simulink model "all_together_simu_v2"  (R2020b)
settings: Solver=FixedStepDiscrete  StartTime=0.0  StopTime=simTime  RelTol=1e-3
InitFcn:
  | setup
values from neighbouring files (symbols this model uses):
  COLS = 752    [setup.m]    (also in setup_old.m = 640)
  Hh = abs(V(:,1)'*sqrt(S(1,1)))    [setup_old.m]
  Hv = abs(U(:,1)*sqrt(S(1,1)))    [setup_old.m]
undefined symbols (not defined in the file or in its folder): gray, Rec, SDTV
libraries: hdlsllib x52, visionhdlio x7, visionsinks x3, simulink x2, visionconversions x1, visionsources x1
(part 1 of 2)
settings Model: DataTypeOverride=Off  SimulationMode=accelerator  Creator=The MathWorks, Inc.  LastModifiedBy=Ethan
settings SolverCC: AutoInsertRateTranBlk=on
settings DataIOCC: LimitDataPoints=on  SaveOutput=off  SignalLogging=off  SaveTime=off  ReturnWorkspaceOutputs=off
settings OptimizationCC: BlockReduction=off  ConditionallyExecuteInputs=off  DefaultParameterBehavior=Inlined  LifeSpan=inf
settings DebuggingCC: AlgebraicLoopMsg=error  SingleTaskRateTransMsg=error  ParameterPrecisionLossMsg=none  AllowSymbolicDim=off  StrictBusMsg=ErrorOnBusTreatedAsVector  SFUnexpectedBacktrackingDiag=warning  SFNoUnconditionalDefaultTransitionDiag=warning  SFExecutionAtInitializationDiag=none  ArithmeticOperatorsInVariantConditions=warning
settings HardwareCC: ProdBitPerPointer=32  ProdBitPerSizeT=32  ProdBitPerPtrDiffT=32  ProdLargestAtomicFloat=None  ProdIntDivRoundTo=Undefined  ProdEndianess=Unspecified  ProdWordSize=32  ProdHWDeviceType=ASIC/FPGA->ASIC/FPGA  ProdEqTarget=off
settings SFSimCC: SimUseLocalCustomCode=off  CustomCodeUndefinedFunction=UseInterfaceOnly
settings RTWCC: RTWUseLocalCustomCode=off
settings CodeAppCC: StateflowObjectComments=on
settings GRTTargetCC: TargetLangStandard=C89/C90 (ANSI)
settings ConfigComp: CovMetricSettings=dw  CovSaveCumulativeToWorkspaceVar=on  CovSaveSingleToWorkspaceVar=on  CovExternalEMLEnable=off  CovSFcnEnable=off

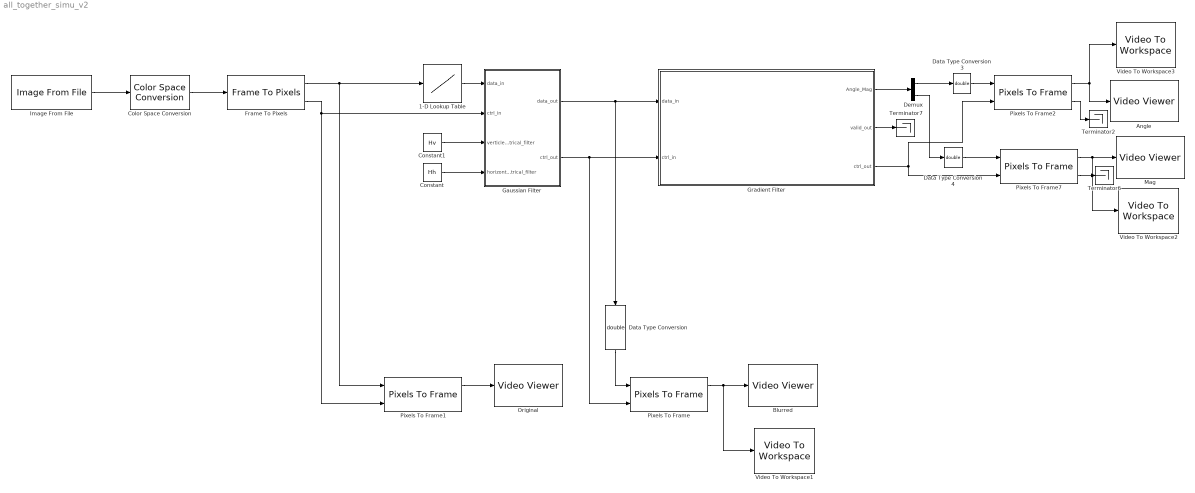
== system all_together_simu_v2 ==
  1-D Lookup Table : Lookup_n-D  NumberOfTableDimensions=1  BreakpointsForDimension1=[0:255]  Table=[0:1/255:1]  ExtrapMethod=Clip  InternalRulePriority=Speed  OutDataTypeStr=fixdt(0,16,15)  RndMeth=Simplest  InputSameDT=on
  Angle : VideoViewer  colormapValue=gray(256)  FigPos=[1922 517 909 409]
  Blurred : VideoViewer  FigPos=[951 815 859 624]
  Color Space Conversion : visionconversions/Color Space  Conversion  conversion=Obsolete  conversionActive=R'G'B' to intensity  wp_str=D65  rec=Rec. 601 (SDTV)  sys=1125/60/2:1  imagePorts=One multidimensional signal
  Constant : Constant  Value=Hh  OutDataTypeStr=Inherit: Inherit via back propagation  SampleTime=-1
  Constant1 : Constant  Value=Hv  OutDataTypeStr=Inherit: Inherit via back propagation  SampleTime=-1
  Data Type Conversion : DataTypeConversion  OutDataTypeStr=double
  Data Type Conversion3 : DataTypeConversion  OutDataTypeStr=double
  Data Type Conversion4 : DataTypeConversion  OutDataTypeStr=double
  Demux : Demux  Outputs=2
  Frame To Pixels : visionhdlio/Frame To Pixels  NumComponents=1  NumPixels=1  VideoFormat=480p  ActivePixelsPerLine=32  ActiveVideoLines=18  TotalPixelsPerLine=42  TotalVideoLines=28  StartingActiveLine=6  FrontPorch=5  SampleTime=0
      settings: SourceProductName=Vision HDL Toolbox
  Gaussian Filter : Subsystem
  Gradient Filter : Subsystem
  Image From File : visionsources/Image From File  Tag=vipblks_nd  FileName=..\..\visualStudio\images\input\start.png  Ts=1  imagePorts=One multidimensional signal  OutPortLabels=R|G|B  ImageDataType=uint8  sdImageDataType=uint(8)  Signed=on  WordLength=16  FractionLengthMode=User-defined  FractionLength=15
  Mag : VideoViewer  FigPos=[1914 1017 954 411]
  Original : VideoViewer  FigPos=[946 1004 813 538]
  Pixels To Frame{,1..2,7} (4 alike) : visionhdlio/Pixels To Frame  NumComponents=1  NumPixels=1  VideoFormat=480p  ActivePixelsPerLine=32  ActiveVideoLines=18  TotalPixelsPerLine=42  TotalVideoLines=28
      settings: SourceProductBaseCode=VT
  Terminator2 : Terminator
  Terminator6 : Terminator
  Terminator7 : Terminator
  Video To Workspace1 : visionsinks/Video To Workspace  VariableName=gaussian  NumInputs=1  DataLimit=10  DecimationFactor=1  LogFi=off  InPortLabels=R|G|B
      settings: SourceProductBaseCode=VP
  Video To Workspace2 : visionsinks/Video To Workspace  VariableName=mag  NumInputs=1  DataLimit=10  DecimationFactor=1  LogFi=off  InPortLabels=R|G|B
      settings: SourceProductBaseCode=VP
  Video To Workspace3 : visionsinks/Video To Workspace  VariableName=angle  NumInputs=1  DataLimit=10  DecimationFactor=1  LogFi=off  InPortLabels=R|G|B
      settings: SourceProductBaseCode=VP
  wires:
  Frame To Pixels/2 -> Pixels To Frame1/2, Gaussian Filter/2(ctrl_in)
  Image From File/1 -> Color Space Conversion/1
  Constant/1 -> Gaussian Filter/4(horizontal_symmetrical_filter)
  Constant1/1 -> Gaussian Filter/3(verticle_symmetrical_filter)
  1-D Lookup Table/1 -> Gaussian Filter/1(data_in)
  Color Space Conversion/1 -> Frame To Pixels/1
  Frame To Pixels/1 -> 1-D Lookup Table/1, Pixels To Frame1/1
  Gaussian Filter/1(data_out) -> Gradient Filter/1(data_in), Data Type Conversion/1
  Gaussian Filter/2(ctrl_out) -> Pixels To Frame/2, Gradient Filter/2(ctrl_in)
  Pixels To Frame/1 -> Video To Workspace1/1, Blurred/1
  Pixels To Frame1/1 -> Original/1
  Pixels To Frame7/1 -> Mag/1, Video To Workspace2/1
  Pixels To Frame2/1 -> Angle/1, Video To Workspace3/1
  Pixels To Frame7/2 -> Terminator6/1
  Pixels To Frame2/2 -> Terminator2/1
  Gradient Filter/1(Angle_Mag) -> Demux/1
  Data Type Conversion3/1 -> Pixels To Frame2/1
  Demux/1 -> Data Type Conversion3/1
  Demux/2 -> Data Type Conversion4/1
  Data Type Conversion4/1 -> Pixels To Frame7/1
  Gradient Filter/3(ctrl_out) -> Pixels To Frame2/2, Pixels To Frame7/2
  Gradient Filter/2(valid_out) -> Terminator7/1
  Data Type Conversion/1 -> Pixels To Frame/1

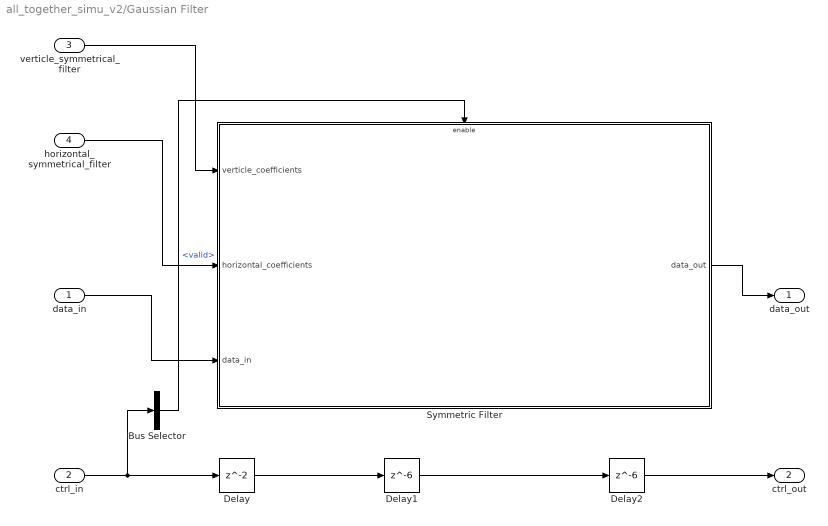
== system all_together_simu_v2/Gaussian Filter ==
  data_in : Inport
  ctrl_in : Inport  Port=2
  verticle_symmetrical_filter : Inport  Port=3
  horizontal_symmetrical_filter : Inport  Port=4
  Bus Selector : BusSelector  OutputSignals=valid
  Delay : Delay
  Delay1 : Delay  DelayLength=6
  Delay2 : Delay  DelayLength=6
  Symmetric Filter : Subsystem
  data_out : Outport
  ctrl_out : Outport  Port=2
  wires:
  ctrl_in/1 -> Bus Selector/1, Delay/1
  Delay/1 -> Delay1/1
  Delay1/1 -> Delay2/1
  Delay2/1 -> ctrl_out/1
  verticle_symmetrical_filter/1 -> Symmetric Filter/1(verticle_coefficients)
  horizontal_symmetrical_filter/1 -> Symmetric Filter/2(horizontal_coefficients)
  data_in/1 -> Symmetric Filter/3(data_in)
  Symmetric Filter/1(data_out) -> data_out/1
  Bus Selector/1 -> Symmetric Filter/Enable  "<valid>"

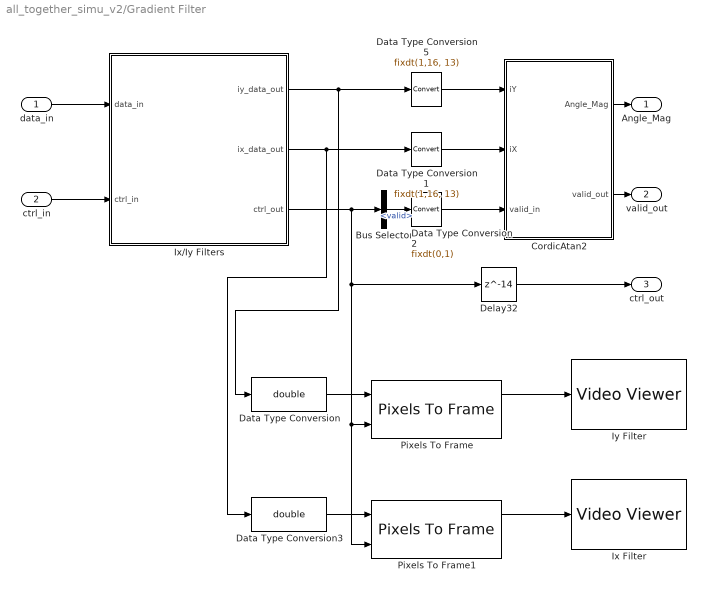
== system all_together_simu_v2/Gradient Filter ==
  data_in : Inport
  ctrl_in : Inport  Port=2
  Bus Selector : BusSelector  OutputSignals=valid
  CordicAtan2 : Subsystem
  Data Type Conversion : DataTypeConversion  OutDataTypeStr=double
  Data Type Conversion1 : DataTypeConversion  OutMin=0  OutMax=1  OutDataTypeStr=fixdt(1,16, 13)
  Data Type Conversion2 : DataTypeConversion  OutMin=0  OutMax=1  OutDataTypeStr=fixdt(0,1)
  Data Type Conversion3 : DataTypeConversion  OutDataTypeStr=double
  Data Type Conversion5 : DataTypeConversion  OutMin=0  OutMax=1  OutDataTypeStr=fixdt(1,16, 13)
  Delay32 : Delay  DelayLength=14
  Ix Filter : VideoViewer  FigPos=[78 822 859 624]
  Ix/Iy Filters : Subsystem
  Iy Filter : VideoViewer  FigPos=[96 1050 859 624]
  Pixels To Frame : visionhdlio/Pixels To Frame  NumComponents=1  NumPixels=1  VideoFormat=480p  ActivePixelsPerLine=32  ActiveVideoLines=18  TotalPixelsPerLine=42  TotalVideoLines=28
      settings: SourceProductBaseCode=VT
  Pixels To Frame1 : visionhdlio/Pixels To Frame  NumComponents=1  NumPixels=1  VideoFormat=480p  ActivePixelsPerLine=32  ActiveVideoLines=18  TotalPixelsPerLine=42  TotalVideoLines=28
      settings: SourceProductBaseCode=VT
  Angle_Mag : Outport
  valid_out : Outport  Port=2
  ctrl_out : Outport  Port=3
  wires:
  CordicAtan2/2(valid_out) -> valid_out/1
  CordicAtan2/1(Angle_Mag) -> Angle_Mag/1
  Ix/Iy Filters/1(iy_data_out) -> Data Type Conversion/1, Data Type Conversion5/1
  Ix/Iy Filters/2(ix_data_out) -> Data Type Conversion3/1, Data Type Conversion1/1
  Data Type Conversion1/1 -> CordicAtan2/2(iX)
  Data Type Conversion2/1 -> CordicAtan2/3(valid_in)
  Ix/Iy Filters/3(ctrl_out) -> Pixels To Frame1/2, Pixels To Frame/2, Delay32/1, Bus Selector/1
  Bus Selector/1 -> Data Type Conversion2/1  "<valid>"
  Data Type Conversion5/1 -> CordicAtan2/1(iY)
  data_in/1 -> Ix/Iy Filters/1(data_in)
  ctrl_in/1 -> Ix/Iy Filters/2(ctrl_in)
  Delay32/1 -> ctrl_out/1
  Pixels To Frame/1 -> Iy Filter/1
  Pixels To Frame1/1 -> Ix Filter/1
  Data Type Conversion/1 -> Pixels To Frame/1
  Data Type Conversion3/1 -> Pixels To Frame1/1

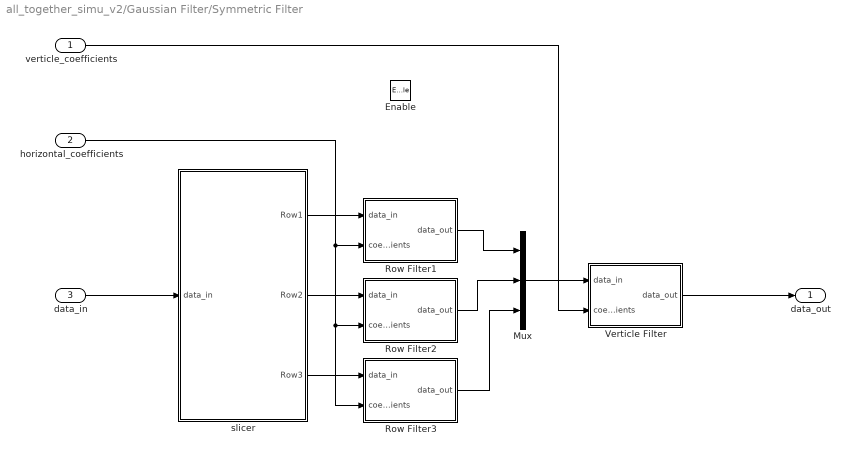
== system all_together_simu_v2/Gaussian Filter/Symmetric Filter ==
  verticle_coefficients : Inport
  horizontal_coefficients : Inport  Port=2
  data_in : Inport  Port=3
  Enable : EnablePort
  Mux : Mux  Inputs=3
  Row Filter1 : Subsystem
  Row Filter2 : Subsystem
  Row Filter3 : Subsystem
  Verticle Filter : Subsystem
  slicer : Subsystem
  data_out : Outport
  wires:
  Row Filter2/1(data_out) -> Mux/2
  Row Filter3/1(data_out) -> Mux/3
  Row Filter1/1(data_out) -> Mux/1
  slicer/1(Row1) -> Row Filter1/1(data_in)
  data_in/1 -> slicer/1(data_in)
  horizontal_coefficients/1 -> Row Filter3/2(coefficients), Row Filter2/2(coefficients), Row Filter1/2(coefficients)
  slicer/2(Row2) -> Row Filter2/1(data_in)
  slicer/3(Row3) -> Row Filter3/1(data_in)
  Mux/1 -> Verticle Filter/1(data_in)
  Verticle Filter/1(data_out) -> data_out/1
  verticle_coefficients/1 -> Verticle Filter/2(coefficients)

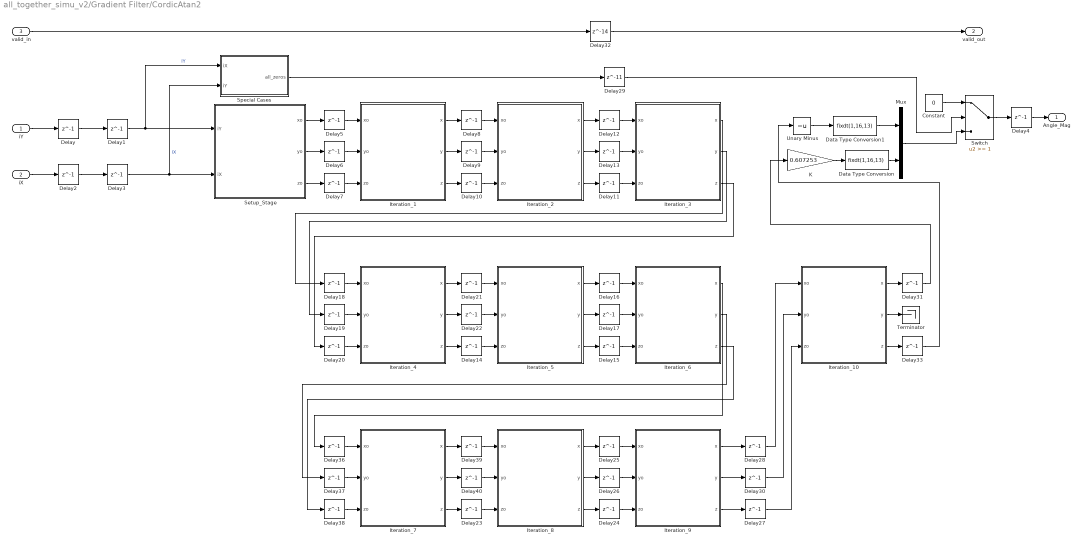
== system all_together_simu_v2/Gradient Filter/CordicAtan2 ==
  iY : Inport
  iX : Inport  Port=2
  valid_in : Inport  Port=3  OutMin=[0]  OutMax=[1]  OutDataTypeStr=fixdt(0,1)
  Constant : Constant  Value=0  OutDataTypeStr=fixdt(1,16,14)  SampleTime=-1
  Data Type Conversion : DataTypeConversion  OutDataTypeStr=fixdt(1,16,13)
  Data Type Conversion1 : DataTypeConversion  OutDataTypeStr=fixdt(1,16,13)
  Delay{,1..28,30..31,33,36..40} (37 alike) : Delay  DelayLength=1
  Delay29 : Delay  DelayLength=11
  Delay32 : Delay  DelayLength=14
  Iteration_1 : Subsystem
  Iteration_10 : Subsystem
  Iteration_2 : Subsystem
  Iteration_3 : Subsystem
  Iteration_4 : Subsystem
  Iteration_5 : Subsystem
  Iteration_6 : Subsystem
  Iteration_7 : Subsystem
  Iteration_8 : Subsystem
  Iteration_9 : Subsystem
  K : Gain  Gain=0.607253  OutDataTypeStr=Inherit: Inherit via back propagation
  Mux : Mux  Inputs=2
  Setup_Stage : Subsystem
  Special Cases : Subsystem
  Switch : Switch  Threshold=1
  Terminator : Terminator
  Unary Minus : UnaryMinus
  Angle_Mag : Outport
  valid_out : Outport  Port=2  OutMin=[0]  OutMax=[1]  OutDataTypeStr=fixdt(0,1)
  wires:
  iY/1 -> Delay/1
  Delay/1 -> Delay1/1
  Delay2/1 -> Delay3/1
  iX/1 -> Delay2/1
  Constant/1 -> Switch/1
  Delay4/1 -> Angle_Mag/1
  Switch/1 -> Delay4/1
  Delay1/1 -> Setup_Stage/1(iY), Special Cases/1(iX)  "iY"
  Delay3/1 -> Special Cases/2(iY), Setup_Stage/2(iX)  "iX"
  Special Cases/1(all_zeros) -> Delay29/1
  Setup_Stage/1(xo) -> Delay5/1
  Setup_Stage/2(yo) -> Delay6/1
  Setup_Stage/3(zo) -> Delay7/1
  Delay7/1 -> Iteration_1/3(zo)
  Delay6/1 -> Iteration_1/2(yo)
  Delay5/1 -> Iteration_1/1(xo)
  Iteration_1/3(z) -> Delay10/1
  Iteration_1/1(x) -> Delay8/1
  Iteration_1/2(y) -> Delay9/1
  Delay9/1 -> Iteration_2/2(yo)
  Delay10/1 -> Iteration_2/3(zo)
  Delay8/1 -> Iteration_2/1(xo)
  Delay11/1 -> Iteration_3/3(zo)
  Delay12/1 -> Iteration_3/1(xo)
  Delay13/1 -> Iteration_3/2(yo)
  Iteration_2/2(y) -> Delay13/1
  Iteration_2/1(x) -> Delay12/1
  Iteration_2/3(z) -> Delay11/1
  Iteration_5/1(x) -> Delay16/1
  Iteration_5/2(y) -> Delay17/1
  Delay16/1 -> Iteration_6/1(xo)
  Delay17/1 -> Iteration_6/2(yo)
  Delay15/1 -> Iteration_6/3(zo)
  Iteration_5/3(z) -> Delay15/1
  Iteration_4/3(z) -> Delay14/1
  Delay14/1 -> Iteration_5/3(zo)
  Iteration_4/2(y) -> Delay22/1
  Delay21/1 -> Iteration_5/1(xo)
  Delay18/1 -> Iteration_4/1(xo)
  Delay20/1 -> Iteration_4/3(zo)
  Iteration_4/1(x) -> Delay21/1
  Delay22/1 -> Iteration_5/2(yo)
  Delay19/1 -> Iteration_4/2(yo)
  Iteration_8/1(x) -> Delay25/1
  Iteration_8/2(y) -> Delay26/1
  Delay25/1 -> Iteration_9/1(xo)
  Delay26/1 -> Iteration_9/2(yo)
  Delay24/1 -> Iteration_9/3(zo)
  Iteration_8/3(z) -> Delay24/1
  Iteration_7/3(z) -> Delay23/1
  Delay23/1 -> Iteration_8/3(zo)
  Iteration_7/2(y) -> Delay40/1
  Delay39/1 -> Iteration_8/1(xo)
  Delay36/1 -> Iteration_7/1(xo)
  Delay38/1 -> Iteration_7/3(zo)
  Iteration_7/1(x) -> Delay39/1
  Delay40/1 -> Iteration_8/2(yo)
  Delay37/1 -> Iteration_7/2(yo)
  Iteration_3/3(z) -> Delay20/1
  Iteration_3/2(y) -> Delay19/1
  Iteration_3/1(x) -> Delay18/1
  Iteration_6/3(z) -> Delay38/1
  Iteration_6/2(y) -> Delay37/1
  Iteration_6/1(x) -> Delay36/1
  Iteration_9/2(y) -> Delay30/1
  Iteration_9/1(x) -> Delay28/1
  Iteration_9/3(z) -> Delay27/1
  Mux/1 -> Switch/3
  Delay29/1 -> Switch/2
  Delay28/1 -> Iteration_10/1(xo)
  Delay30/1 -> Iteration_10/2(yo)
  Delay27/1 -> Iteration_10/3(zo)
  Iteration_10/1(x) -> Delay31/1
  Delay31/1 -> K/1
  Iteration_10/2(y) -> Terminator/1
  Iteration_10/3(z) -> Delay33/1
  Delay33/1 -> Unary Minus/1
  Unary Minus/1 -> Data Type Conversion1/1
  valid_in/1 -> Delay32/1
  Delay32/1 -> valid_out/1
  Data Type Conversion/1 -> Mux/2
  K/1 -> Data Type Conversion/1
  Data Type Conversion1/1 -> Mux/1

== system all_together_simu_v2/Gradient Filter/Ix//Iy Filters ==
  data_in : Inport
  ctrl_in : Inport  Port=2
  Delay : Delay
  Delay1 : Delay
  Delay2 : Delay
  Ix Filter : Subsystem
  Iy Filter : Subsystem
  iy_data_out : Outport
  ix_data_out : Outport  Port=2
  ctrl_out : Outport  Port=3
  wires:
  ctrl_in/1 -> Iy Filter/2(ctrl_in), Ix Filter/2(ctrl_in), Delay/1
  Iy Filter/1(data_out) -> iy_data_out/1
  data_in/1 -> Iy Filter/1(data_in), Ix Filter/1(data_in)
  Delay2/1 -> ctrl_out/1
  Delay1/1 -> Delay2/1
  Delay/1 -> Delay1/1
  Ix Filter/1(data_out) -> ix_data_out/1

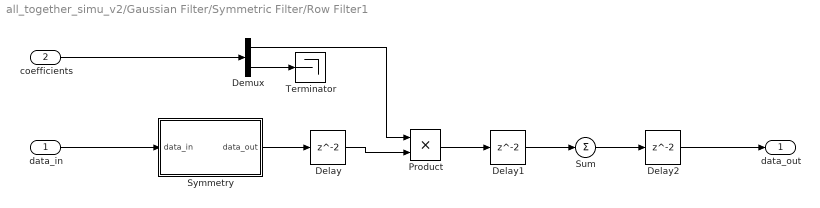
== system all_together_simu_v2/Gaussian Filter/Symmetric Filter/Row Filter1 ==
  data_in : Inport
  coefficients : Inport  Port=2
  Delay : Delay
  Delay1 : Delay
  Delay2 : Delay
  Demux : Demux  Outputs=[2, 1]
  Product : Product
  Sum : Sum  Inputs=1  OutDataTypeStr=Inherit: Same as accumulator
  Symmetry : Subsystem
  Terminator : Terminator
  data_out : Outport
  wires:
  Product/1 -> Delay1/1
  Symmetry/1(data_out) -> Delay/1
  Delay/1 -> Product/2
  Delay1/1 -> Sum/1
  Delay2/1 -> data_out/1
  Sum/1 -> Delay2/1
  data_in/1 -> Symmetry/1(data_in)
  coefficients/1 -> Demux/1
  Demux/1 -> Product/1
  Demux/2 -> Terminator/1

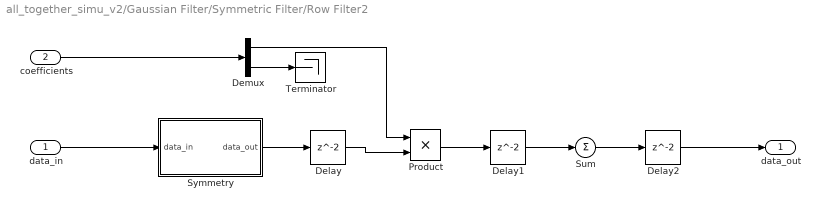
== system all_together_simu_v2/Gaussian Filter/Symmetric Filter/Row Filter2 ==
  data_in : Inport
  coefficients : Inport  Port=2
  Delay : Delay
  Delay1 : Delay
  Delay2 : Delay
  Demux : Demux  Outputs=[2, 1]
  Product : Product
  Sum : Sum  Inputs=1  OutDataTypeStr=Inherit: Same as accumulator
  Symmetry : Subsystem
  Terminator : Terminator
  data_out : Outport
  wires:
  Product/1 -> Delay1/1
  Symmetry/1(data_out) -> Delay/1
  Delay/1 -> Product/2
  Delay1/1 -> Sum/1
  Delay2/1 -> data_out/1
  Sum/1 -> Delay2/1
  data_in/1 -> Symmetry/1(data_in)
  coefficients/1 -> Demux/1
  Demux/1 -> Product/1
  Demux/2 -> Terminator/1

== system all_together_simu_v2/Gaussian Filter/Symmetric Filter/Row Filter3 ==
  data_in : Inport
  coefficients : Inport  Port=2
  Delay : Delay
  Delay1 : Delay
  Delay2 : Delay
  Demux : Demux  Outputs=[2, 1]
  Product : Product
  Sum : Sum  Inputs=1  OutDataTypeStr=Inherit: Same as accumulator
  Symmetry : Subsystem
  Terminator : Terminator
  data_out : Outport
  wires:
  Product/1 -> Delay1/1
  Symmetry/1(data_out) -> Delay/1
  Delay/1 -> Product/2
  Delay1/1 -> Sum/1
  Delay2/1 -> data_out/1
  Sum/1 -> Delay2/1
  data_in/1 -> Symmetry/1(data_in)
  coefficients/1 -> Demux/1
  Demux/1 -> Product/1
  Demux/2 -> Terminator/1

== system all_together_simu_v2/Gaussian Filter/Symmetric Filter/Verticle Filter ==
  data_in : Inport
  coefficients : Inport  Port=2
  Delay : Delay
  Delay1 : Delay
  Delay2 : Delay
  Demux : Demux  Outputs=[2, 1]
  Product : Product
  Sum : Sum  Inputs=1  OutDataTypeStr=Inherit: Same as accumulator
  Symmetry : Subsystem
  Terminator : Terminator
  data_out : Outport
  wires:
  Product/1 -> Delay1/1
  Symmetry/1(data_out) -> Delay/1
  Delay/1 -> Product/2
  Delay1/1 -> Sum/1
  Delay2/1 -> data_out/1
  Sum/1 -> Delay2/1
  data_in/1 -> Symmetry/1(data_in)
  coefficients/1 -> Demux/1
  Demux/1 -> Product/1
  Demux/2 -> Terminator/1

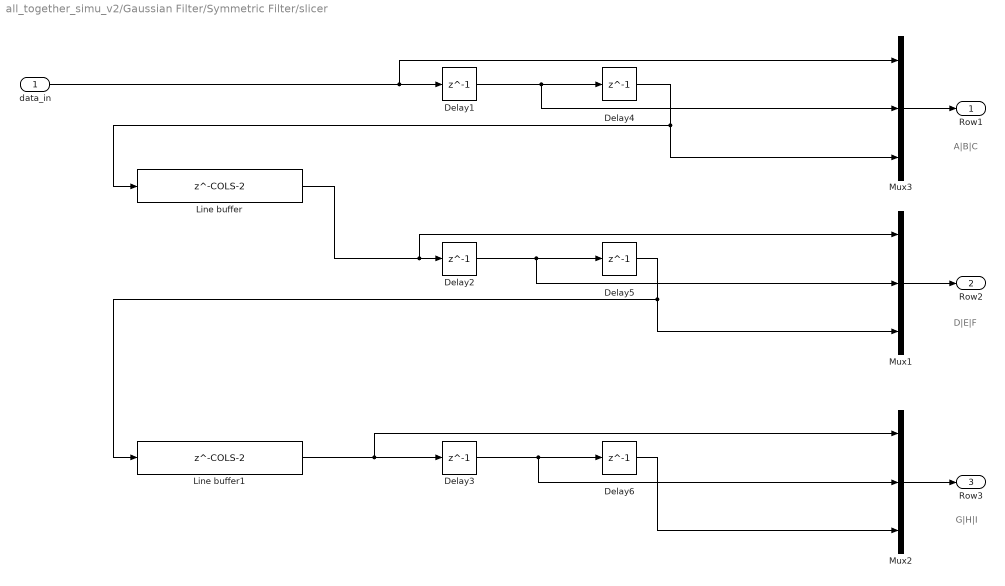
== system all_together_simu_v2/Gaussian Filter/Symmetric Filter/slicer ==
  note: A|B|C
  note: D|E|F
  note: G|H|I
  data_in : Inport
  Delay{1..6} (6 alike) : Delay  DelayLength=1  InitialCondition=0
  Line buffer : Delay  DelayLength=COLS-2  InitialCondition=0
  Line buffer1 : Delay  DelayLength=COLS-2  InitialCondition=0
  Mux1 : Mux  Inputs=3
  Mux2 : Mux  Inputs=3
  Mux3 : Mux  Inputs=3
  Row1 : Outport  VectorParamsAs1DForOutWhenUnconnected=off
  Row2 : Outport  Port=2  VectorParamsAs1DForOutWhenUnconnected=off
  Row3 : Outport  Port=3  VectorParamsAs1DForOutWhenUnconnected=off
  wires:
  Delay4/1 -> Mux3/3, Line buffer/1
  data_in/1 -> Mux3/1, Delay1/1
  Delay1/1 -> Mux3/2, Delay4/1
  Delay3/1 -> Mux2/2, Delay6/1
  Delay5/1 -> Mux1/3, Line buffer1/1
  Delay6/1 -> Mux2/3
  Line buffer/1 -> Mux1/1, Delay2/1
  Line buffer1/1 -> Mux2/1, Delay3/1
  Delay2/1 -> Mux1/2, Delay5/1
  Mux1/1 -> Row2/1
  Mux2/1 -> Row3/1
  Mux3/1 -> Row1/1

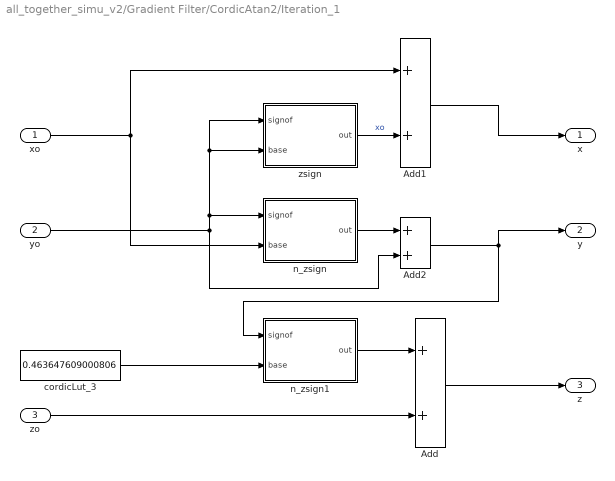
== system all_together_simu_v2/Gradient Filter/CordicAtan2/Iteration_1 ==
  xo : Inport
  yo : Inport  Port=2
  zo : Inport  Port=3
  Add : Sum
  Add1 : Sum
  Add2 : Sum
  cordicLut_3 : Constant  Value=0.463647609000806  OutDataTypeStr=fixdt(1,16,16)  SampleTime=-1
  n_zsign : Subsystem
  n_zsign1 : Subsystem
  zsign : Subsystem
  x : Outport
  y : Outport  Port=2
  z : Outport  Port=3
  wires:
  Add/1 -> z/1
  cordicLut_3/1 -> n_zsign1/2(base)
  zo/1 -> Add/2
  n_zsign1/1(out) -> Add/1
  yo/1 -> zsign/2(base), zsign/1(signof), n_zsign/1(signof), Add2/2
  zsign/1(out) -> Add1/2  "xo"
  xo/1 -> n_zsign/2(base), Add1/1
  Add1/1 -> x/1
  n_zsign/1(out) -> Add2/1
  Add2/1 -> n_zsign1/1(signof), y/1

== system all_together_simu_v2/Gradient Filter/CordicAtan2/Iteration_10 ==
  xo : Inport
  yo : Inport  Port=2
  zo : Inport  Port=3
  Add : Sum
  X_Logic : Subsystem
  Y_Logic : Subsystem
  cordicLut_12 : Constant  Value=0.000976562189559320  OutDataTypeStr=fixdt(1,16,24)  SampleTime=-1
  n_zsign : Subsystem
  x : Outport
  y : Outport  Port=2
  z : Outport  Port=3
  wires:
  Add/1 -> z/1
  cordicLut_12/1 -> n_zsign/2(base)
  zo/1 -> Add/2
  n_zsign/1(out) -> Add/1
  yo/1 -> Y_Logic/2(yo), X_Logic/2(yo)
  xo/1 -> Y_Logic/1(xo), X_Logic/1(xo)
  X_Logic/1(x) -> x/1
  Y_Logic/1(y) -> n_zsign/1(signof), y/1

== system all_together_simu_v2/Gradient Filter/CordicAtan2/Iteration_2 ==
  xo : Inport
  yo : Inport  Port=2
  zo : Inport  Port=3
  Add : Sum
  X_Logic : Subsystem
  Y_Logic : Subsystem
  cordicLut_4 : Constant  Value=0.244978663126864  OutDataTypeStr=fixdt(1,16, 17)  SampleTime=-1
  n_zsign : Subsystem
  x : Outport
  y : Outport  Port=2
  z : Outport  Port=3
  wires:
  Add/1 -> z/1
  cordicLut_4/1 -> n_zsign/2(base)
  zo/1 -> Add/2
  n_zsign/1(out) -> Add/1
  yo/1 -> Y_Logic/2(yo), X_Logic/2(yo)
  xo/1 -> Y_Logic/1(xo), X_Logic/1(xo)
  X_Logic/1(x) -> x/1
  Y_Logic/1(y) -> n_zsign/1(signof), y/1

== system all_together_simu_v2/Gradient Filter/CordicAtan2/Iteration_3 ==
  xo : Inport
  yo : Inport  Port=2
  zo : Inport  Port=3
  Add : Sum
  X_Logic : Subsystem
  Y_Logic : Subsystem
  cordicLut_5 : Constant  Value=0.124354994546761  OutDataTypeStr=fixdt(1,16,17)  SampleTime=-1
  n_zsign : Subsystem
  x : Outport
  y : Outport  Port=2
  z : Outport  Port=3
  wires:
  Add/1 -> z/1
  cordicLut_5/1 -> n_zsign/2(base)
  zo/1 -> Add/2
  n_zsign/1(out) -> Add/1
  yo/1 -> Y_Logic/2(yo), X_Logic/2(yo)
  xo/1 -> Y_Logic/1(xo), X_Logic/1(xo)
  X_Logic/1(x) -> x/1
  Y_Logic/1(y) -> n_zsign/1(signof), y/1

== system all_together_simu_v2/Gradient Filter/CordicAtan2/Iteration_4 ==
  xo : Inport
  yo : Inport  Port=2
  zo : Inport  Port=3
  Add : Sum
  X_Logic : Subsystem
  Y_Logic : Subsystem
  cordicLut_6 : Constant  Value=0.0624188099959574  OutDataTypeStr=fixdt(1,16,18)  SampleTime=-1
  n_zsign : Subsystem
  x : Outport
  y : Outport  Port=2
  z : Outport  Port=3
  wires:
  Add/1 -> z/1
  cordicLut_6/1 -> n_zsign/2(base)
  zo/1 -> Add/2
  n_zsign/1(out) -> Add/1
  yo/1 -> Y_Logic/2(yo), X_Logic/2(yo)
  xo/1 -> Y_Logic/1(xo), X_Logic/1(xo)
  X_Logic/1(x) -> x/1
  Y_Logic/1(y) -> n_zsign/1(signof), y/1

== system all_together_simu_v2/Gradient Filter/CordicAtan2/Iteration_5 ==
  xo : Inport
  yo : Inport  Port=2
  zo : Inport  Port=3
  Add : Sum
  X_Logic : Subsystem
  Y_Logic : Subsystem
  cordicLut_7 : Constant  Value=0.0312398334302683  OutDataTypeStr=fixdt(1,16,19)  SampleTime=-1
  n_zsign : Subsystem
  x : Outport
  y : Outport  Port=2
  z : Outport  Port=3
  wires:
  Add/1 -> z/1
  cordicLut_7/1 -> n_zsign/2(base)
  zo/1 -> Add/2
  n_zsign/1(out) -> Add/1
  yo/1 -> Y_Logic/2(yo), X_Logic/2(yo)
  xo/1 -> Y_Logic/1(xo), X_Logic/1(xo)
  X_Logic/1(x) -> x/1
  Y_Logic/1(y) -> n_zsign/1(signof), y/1

== system all_together_simu_v2/Gradient Filter/CordicAtan2/Iteration_6 ==
  xo : Inport
  yo : Inport  Port=2
  zo : Inport  Port=3
  Add : Sum
  X_Logic : Subsystem
  Y_Logic : Subsystem
  cordicLut_8 : Constant  Value=0.0156237286204768  OutDataTypeStr=fixdt(1,16,20)  SampleTime=-1
  n_zsign : Subsystem
  x : Outport
  y : Outport  Port=2
  z : Outport  Port=3
  wires:
  Add/1 -> z/1
  cordicLut_8/1 -> n_zsign/2(base)
  zo/1 -> Add/2
  n_zsign/1(out) -> Add/1
  yo/1 -> Y_Logic/2(yo), X_Logic/2(yo)
  xo/1 -> Y_Logic/1(xo), X_Logic/1(xo)
  X_Logic/1(x) -> x/1
  Y_Logic/1(y) -> n_zsign/1(signof), y/1

== system all_together_simu_v2/Gradient Filter/CordicAtan2/Iteration_7 ==
  xo : Inport
  yo : Inport  Port=2
  zo : Inport  Port=3
  Add : Sum
  X_Logic : Subsystem
  Y_Logic : Subsystem
  cordicLut_9 : Constant  Value=0.00781234106010111  OutDataTypeStr=fixdt(1,16,21)  SampleTime=-1
  n_zsign : Subsystem
  x : Outport
  y : Outport  Port=2
  z : Outport  Port=3
  wires:
  Add/1 -> z/1
  cordicLut_9/1 -> n_zsign/2(base)
  zo/1 -> Add/2
  n_zsign/1(out) -> Add/1
  yo/1 -> Y_Logic/2(yo), X_Logic/2(yo)
  xo/1 -> Y_Logic/1(xo), X_Logic/1(xo)
  X_Logic/1(x) -> x/1
  Y_Logic/1(y) -> n_zsign/1(signof), y/1

== system all_together_simu_v2/Gradient Filter/CordicAtan2/Iteration_8 ==
  xo : Inport
  yo : Inport  Port=2
  zo : Inport  Port=3
  Add : Sum
  X_Logic : Subsystem
  Y_Logic : Subsystem
  cordicLut_10 : Constant  Value=0.00390623013196697  OutDataTypeStr=fixdt(1,16,22)  SampleTime=-1
  n_zsign : Subsystem
  x : Outport
  y : Outport  Port=2
  z : Outport  Port=3
  wires:
  Add/1 -> z/1
  cordicLut_10/1 -> n_zsign/2(base)
  zo/1 -> Add/2
  n_zsign/1(out) -> Add/1
  yo/1 -> Y_Logic/2(yo), X_Logic/2(yo)
  xo/1 -> Y_Logic/1(xo), X_Logic/1(xo)
  X_Logic/1(x) -> x/1
  Y_Logic/1(y) -> n_zsign/1(signof), y/1

== system all_together_simu_v2/Gradient Filter/CordicAtan2/Iteration_9 ==
  xo : Inport
  yo : Inport  Port=2
  zo : Inport  Port=3
  Add : Sum
  X_Logic : Subsystem
  Y_Logic : Subsystem
  cordicLut_11 : Constant  Value=0.00195312251647882  OutDataTypeStr=fixdt(1,16,23)  SampleTime=-1
  n_zsign : Subsystem
  x : Outport
  y : Outport  Port=2
  z : Outport  Port=3
  wires:
  Add/1 -> z/1
  cordicLut_11/1 -> n_zsign/2(base)
  zo/1 -> Add/2
  n_zsign/1(out) -> Add/1
  yo/1 -> Y_Logic/2(yo), X_Logic/2(yo)
  xo/1 -> Y_Logic/1(xo), X_Logic/1(xo)
  X_Logic/1(x) -> x/1
  Y_Logic/1(y) -> n_zsign/1(signof), y/1

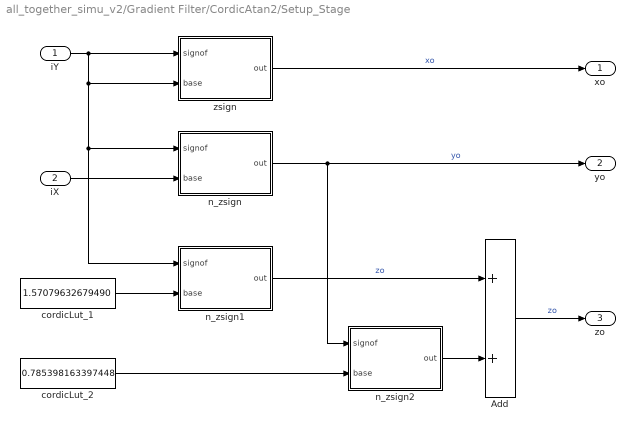
== system all_together_simu_v2/Gradient Filter/CordicAtan2/Setup_Stage ==
  iY : Inport
  iX : Inport  Port=2
  Add : Sum
  cordicLut_1 : Constant  Value=1.57079632679490  OutDataTypeStr=fixdt(1,16, 14)  SampleTime=-1
  cordicLut_2 : Constant  Value=0.785398163397448  OutDataTypeStr=fixdt(1,16, 15)  SampleTime=-1
  n_zsign : Subsystem
  n_zsign1 : Subsystem
  n_zsign2 : Subsystem
  zsign : Subsystem
  xo : Outport
  yo : Outport  Port=2
  zo : Outport  Port=3
  wires:
  cordicLut_1/1 -> n_zsign1/2(base)
  iY/1 -> zsign/2(base), n_zsign1/1(signof), n_zsign/1(signof), zsign/1(signof)
  n_zsign/1(out) -> n_zsign2/1(signof), yo/1  "yo"
  n_zsign1/1(out) -> Add/1  "zo"
  cordicLut_2/1 -> n_zsign2/2(base)
  iX/1 -> n_zsign/2(base)
  n_zsign2/1(out) -> Add/2
  Add/1 -> zo/1  "zo"
  zsign/1(out) -> xo/1  "xo"

== system all_together_simu_v2/Gradient Filter/CordicAtan2/Special Cases ==
  iX : Inport
  iY : Inport  Port=2
  Compare To Zero : simulink/Logic and Bit Operations/Compare To Zero  relop===  OutDataTypeStr=boolean
  Compare To Zero1 : simulink/Logic and Bit Operations/Compare To Zero  relop===  OutDataTypeStr=boolean
  Logical Operator : Logic  AllPortsSameDT=off  OutDataTypeStr=boolean
  all_zeros : Outport
  wires:
  Compare To Zero1/1 -> Logical Operator/2
  Logical Operator/1 -> all_zeros/1
  iY/1 -> Compare To Zero1/1
  Compare To Zero/1 -> Logical Operator/1
  iX/1 -> Compare To Zero/1

== system all_together_simu_v2/Gradient Filter/Ix//Iy Filters/Ix Filter ==
  data_in : Inport
  ctrl_in : Inport  Port=2
  Bus Selector : BusSelector  OutputSignals=valid
  Filter : Subsystem
  data_out : Outport
  wires:
  ctrl_in/1 -> Bus Selector/1
  data_in/1 -> Filter/1(data_in)
  Filter/1(data_out) -> data_out/1
  Bus Selector/1 -> Filter/Enable  "<valid>"

== system all_together_simu_v2/Gradient Filter/Ix//Iy Filters/Iy Filter ==
  data_in : Inport
  ctrl_in : Inport  Port=2
  Bus Selector : BusSelector  OutputSignals=valid
  Filter : Subsystem
  data_out : Outport
  wires:
  ctrl_in/1 -> Bus Selector/1
  data_in/1 -> Filter/1(data_in)
  Filter/1(data_out) -> data_out/1
  Bus Selector/1 -> Filter/Enable  "<valid>"

== system all_together_simu_v2/Gaussian Filter/Symmetric Filter/Row Filter1/Symmetry ==
  data_in : Inport
  Data Type Duplicate : DataTypeDuplicate
  Data Type Conversion1 : DataTypeConversion
  Demux : Demux  Outputs=3
  Mux : Mux  Inputs=2
  Sum3 : Sum  Inputs=|++
  data_out : Outport
  wires:
  Data Type Conversion1/1 -> Data Type Duplicate/2, Mux/2
  Sum3/1 -> Mux/1, Data Type Duplicate/1
  data_in/1 -> Demux/1
  Demux/2 -> Data Type Conversion1/1
  Demux/3 -> Sum3/2
  Demux/1 -> Sum3/1
  Mux/1 -> data_out/1

== system all_together_simu_v2/Gaussian Filter/Symmetric Filter/Row Filter2/Symmetry ==
  data_in : Inport
  Data Type Duplicate : DataTypeDuplicate
  Data Type Conversion1 : DataTypeConversion
  Demux : Demux  Outputs=3
  Mux : Mux  Inputs=2
  Sum3 : Sum  Inputs=|++
  data_out : Outport
  wires:
  Data Type Conversion1/1 -> Data Type Duplicate/2, Mux/2
  Sum3/1 -> Mux/1, Data Type Duplicate/1
  data_in/1 -> Demux/1
  Demux/2 -> Data Type Conversion1/1
  Demux/3 -> Sum3/2
  Demux/1 -> Sum3/1
  Mux/1 -> data_out/1

== system all_together_simu_v2/Gaussian Filter/Symmetric Filter/Row Filter3/Symmetry ==
  data_in : Inport
  Data Type Duplicate : DataTypeDuplicate
  Data Type Conversion1 : DataTypeConversion
  Demux : Demux  Outputs=3
  Mux : Mux  Inputs=2
  Sum3 : Sum  Inputs=|++
  data_out : Outport
  wires:
  Data Type Conversion1/1 -> Data Type Duplicate/2, Mux/2
  Sum3/1 -> Mux/1, Data Type Duplicate/1
  data_in/1 -> Demux/1
  Demux/2 -> Data Type Conversion1/1
  Demux/3 -> Sum3/2
  Demux/1 -> Sum3/1
  Mux/1 -> data_out/1

== system all_together_simu_v2/Gaussian Filter/Symmetric Filter/Verticle Filter/Symmetry ==
  data_in : Inport
  Data Type Duplicate : DataTypeDuplicate
  Data Type Conversion1 : DataTypeConversion
  Demux : Demux  Outputs=3
  Mux : Mux  Inputs=2
  Sum3 : Sum  Inputs=|++
  data_out : Outport
  wires:
  Data Type Conversion1/1 -> Data Type Duplicate/2, Mux/2
  Sum3/1 -> Mux/1, Data Type Duplicate/1
  data_in/1 -> Demux/1
  Demux/2 -> Data Type Conversion1/1
  Demux/3 -> Sum3/2
  Demux/1 -> Sum3/1
  Mux/1 -> data_out/1

== system all_together_simu_v2/Gradient Filter/CordicAtan2/Iteration_1/n_zsign ==
  signof : Inport
  base : Inport  Port=2
  Bit Slice : hdlsllib/Logic and Bit Operations/Bit Slice  lidx=15  ridx=15
      settings: SourceProductBaseCode=SL
  Switch : Switch  Criteria=u2 > Threshold
  Unary Minus : UnaryMinus
  out : Outport
  wires:
  Bit Slice/1 -> Switch/2
  signof/1 -> Bit Slice/1
  base/1 -> Switch/1, Unary Minus/1
  Switch/1 -> out/1
  Unary Minus/1 -> Switch/3

== system all_together_simu_v2/Gradient Filter/CordicAtan2/Iteration_1/n_zsign1 ==
  signof : Inport
  base : Inport  Port=2
  Bit Slice : hdlsllib/Logic and Bit Operations/Bit Slice  lidx=15  ridx=15
      settings: SourceProductBaseCode=SL
  Switch : Switch  Criteria=u2 > Threshold
  Unary Minus : UnaryMinus
  out : Outport
  wires:
  Bit Slice/1 -> Switch/2
  signof/1 -> Bit Slice/1
  base/1 -> Switch/1, Unary Minus/1
  Switch/1 -> out/1
  Unary Minus/1 -> Switch/3

== system all_together_simu_v2/Gradient Filter/CordicAtan2/Iteration_1/zsign ==
  signof : Inport
  base : Inport  Port=2
  Bit Slice : hdlsllib/Logic and Bit Operations/Bit Slice  lidx=15  ridx=15
      settings: SourceProductBaseCode=SL
  Switch : Switch  Criteria=u2 > Threshold
  Unary Minus : UnaryMinus
  out : Outport
  wires:
  signof/1 -> Bit Slice/1
  Bit Slice/1 -> Switch/2
  base/1 -> Switch/3, Unary Minus/1
  Switch/1 -> out/1
  Unary Minus/1 -> Switch/1

== system all_together_simu_v2/Gradient Filter/CordicAtan2/Iteration_10/X_Logic ==
  xo : Inport
  yo : Inport  Port=2
  Add2 : Sum
  Bit Shift : hdlsllib/Logic and Bit Operations/Bit Shift  mode=Shift Right Arithmetic  N=9
  zsign : Subsystem
  x : Outport
  wires:
  yo/1 -> zsign/1(signof), Bit Shift/1
  Bit Shift/1 -> zsign/2(base)
  xo/1 -> Add2/1
  Add2/1 -> x/1
  zsign/1(out) -> Add2/2  "xo"

== system all_together_simu_v2/Gradient Filter/CordicAtan2/Iteration_10/Y_Logic ==
  xo : Inport
  yo : Inport  Port=2
  Add1 : Sum  OutDataTypeStr=fixdt(1,16,21)
  Bit Shift : hdlsllib/Logic and Bit Operations/Bit Shift  mode=Shift Right Arithmetic  N=9
  n_zsign : Subsystem
  y : Outport
  wires:
  Bit Shift/1 -> n_zsign/2(base)
  n_zsign/1(out) -> Add1/2
  Add1/1 -> y/1
  xo/1 -> Bit Shift/1
  yo/1 -> n_zsign/1(signof), Add1/1

== system all_together_simu_v2/Gradient Filter/CordicAtan2/Iteration_10/n_zsign ==
  signof : Inport
  base : Inport  Port=2
  Bit Slice : hdlsllib/Logic and Bit Operations/Bit Slice  lidx=15  ridx=15
      settings: SourceProductBaseCode=SL
  Switch : Switch  Criteria=u2 > Threshold
  Unary Minus : UnaryMinus
  out : Outport
  wires:
  Bit Slice/1 -> Switch/2
  signof/1 -> Bit Slice/1
  base/1 -> Switch/1, Unary Minus/1
  Switch/1 -> out/1
  Unary Minus/1 -> Switch/3

== system all_together_simu_v2/Gradient Filter/CordicAtan2/Iteration_2/X_Logic ==
  xo : Inport
  yo : Inport  Port=2
  Add2 : Sum
  Bit Shift : hdlsllib/Logic and Bit Operations/Bit Shift  mode=Shift Right Arithmetic  N=1
  zsign1 : Subsystem
  x : Outport
  wires:
  yo/1 -> zsign1/1(signof), Bit Shift/1
  Bit Shift/1 -> zsign1/2(base)
  xo/1 -> Add2/1
  Add2/1 -> x/1
  zsign1/1(out) -> Add2/2  "xo"

== system all_together_simu_v2/Gradient Filter/CordicAtan2/Iteration_2/Y_Logic ==
  xo : Inport
  yo : Inport  Port=2
  Add1 : Sum
  Bit Shift : hdlsllib/Logic and Bit Operations/Bit Shift  mode=Shift Right Arithmetic  N=1
  n_zsign : Subsystem
  y : Outport
  wires:
  Bit Shift/1 -> n_zsign/2(base)
  n_zsign/1(out) -> Add1/2
  Add1/1 -> y/1
  xo/1 -> Bit Shift/1
  yo/1 -> n_zsign/1(signof), Add1/1

== system all_together_simu_v2/Gradient Filter/CordicAtan2/Iteration_2/n_zsign ==
  signof : Inport
  base : Inport  Port=2
  Bit Slice : hdlsllib/Logic and Bit Operations/Bit Slice  lidx=15  ridx=15
      settings: SourceProductBaseCode=SL
  Switch : Switch  Criteria=u2 > Threshold
  Unary Minus : UnaryMinus
  out : Outport
  wires:
  Bit Slice/1 -> Switch/2
  signof/1 -> Bit Slice/1
  base/1 -> Switch/1, Unary Minus/1
  Switch/1 -> out/1
  Unary Minus/1 -> Switch/3

== system all_together_simu_v2/Gradient Filter/CordicAtan2/Iteration_3/X_Logic ==
  xo : Inport
  yo : Inport  Port=2
  Add2 : Sum
  Bit Shift : hdlsllib/Logic and Bit Operations/Bit Shift  mode=Shift Right Arithmetic  N=2
  zsign : Subsystem
  x : Outport
  wires:
  yo/1 -> zsign/1(signof), Bit Shift/1
  Bit Shift/1 -> zsign/2(base)
  xo/1 -> Add2/1
  Add2/1 -> x/1
  zsign/1(out) -> Add2/2  "xo"

== system all_together_simu_v2/Gradient Filter/CordicAtan2/Iteration_3/Y_Logic ==
  xo : Inport
  yo : Inport  Port=2
  Add1 : Sum  OutDataTypeStr=fixdt(1,16,15)
  Bit Shift : hdlsllib/Logic and Bit Operations/Bit Shift  mode=Shift Right Arithmetic  N=2
  n_zsign : Subsystem
  y : Outport
  wires:
  Bit Shift/1 -> n_zsign/2(base)
  n_zsign/1(out) -> Add1/2
  Add1/1 -> y/1
  xo/1 -> Bit Shift/1
  yo/1 -> n_zsign/1(signof), Add1/1

== system all_together_simu_v2/Gradient Filter/CordicAtan2/Iteration_3/n_zsign ==
  signof : Inport
  base : Inport  Port=2
  Bit Slice : hdlsllib/Logic and Bit Operations/Bit Slice  lidx=15  ridx=15
      settings: SourceProductBaseCode=SL
  Switch : Switch  Criteria=u2 > Threshold
  Unary Minus : UnaryMinus
  out : Outport
  wires:
  Bit Slice/1 -> Switch/2
  signof/1 -> Bit Slice/1
  base/1 -> Switch/1, Unary Minus/1
  Switch/1 -> out/1
  Unary Minus/1 -> Switch/3

== system all_together_simu_v2/Gradient Filter/CordicAtan2/Iteration_4/X_Logic ==
  xo : Inport
  yo : Inport  Port=2
  Add2 : Sum
  Bit Shift : hdlsllib/Logic and Bit Operations/Bit Shift  mode=Shift Right Arithmetic  N=3
  zsign : Subsystem
  x : Outport
  wires:
  yo/1 -> zsign/1(signof), Bit Shift/1
  Bit Shift/1 -> zsign/2(base)
  xo/1 -> Add2/1
  Add2/1 -> x/1
  zsign/1(out) -> Add2/2  "xo"

== system all_together_simu_v2/Gradient Filter/CordicAtan2/Iteration_4/Y_Logic ==
  xo : Inport
  yo : Inport  Port=2
  Add1 : Sum  OutDataTypeStr=fixdt(1,16,16)
  Bit Shift : hdlsllib/Logic and Bit Operations/Bit Shift  mode=Shift Right Arithmetic  N=3
  n_zsign : Subsystem
  y : Outport
  wires:
  Bit Shift/1 -> n_zsign/2(base)
  n_zsign/1(out) -> Add1/2
  Add1/1 -> y/1
  xo/1 -> Bit Shift/1
  yo/1 -> n_zsign/1(signof), Add1/1

== system all_together_simu_v2/Gradient Filter/CordicAtan2/Iteration_4/n_zsign ==
  signof : Inport
  base : Inport  Port=2
  Bit Slice : hdlsllib/Logic and Bit Operations/Bit Slice  lidx=15  ridx=15
      settings: SourceProductBaseCode=SL
  Switch : Switch  Criteria=u2 > Threshold
  Unary Minus : UnaryMinus
  out : Outport
  wires:
  Bit Slice/1 -> Switch/2
  signof/1 -> Bit Slice/1
  base/1 -> Switch/1, Unary Minus/1
  Switch/1 -> out/1
  Unary Minus/1 -> Switch/3

== system all_together_simu_v2/Gradient Filter/CordicAtan2/Iteration_5/X_Logic ==
  xo : Inport
  yo : Inport  Port=2
  Add2 : Sum
  Bit Shift : hdlsllib/Logic and Bit Operations/Bit Shift  mode=Shift Right Arithmetic  N=4
  zsign : Subsystem
  x : Outport
  wires:
  yo/1 -> zsign/1(signof), Bit Shift/1
  Bit Shift/1 -> zsign/2(base)
  xo/1 -> Add2/1
  Add2/1 -> x/1
  zsign/1(out) -> Add2/2  "xo"

== system all_together_simu_v2/Gradient Filter/CordicAtan2/Iteration_5/Y_Logic ==
  xo : Inport
  yo : Inport  Port=2
  Add1 : Sum  OutDataTypeStr=fixdt(1,16,18)
  Bit Shift : hdlsllib/Logic and Bit Operations/Bit Shift  mode=Shift Right Arithmetic  N=4
  n_zsign : Subsystem
  y : Outport
  wires:
  Bit Shift/1 -> n_zsign/2(base)
  n_zsign/1(out) -> Add1/2
  Add1/1 -> y/1
  xo/1 -> Bit Shift/1
  yo/1 -> n_zsign/1(signof), Add1/1

== system all_together_simu_v2/Gradient Filter/CordicAtan2/Iteration_5/n_zsign ==
  signof : Inport
  base : Inport  Port=2
  Bit Slice : hdlsllib/Logic and Bit Operations/Bit Slice  lidx=15  ridx=15
      settings: SourceProductBaseCode=SL
  Switch : Switch  Criteria=u2 > Threshold
  Unary Minus : UnaryMinus
  out : Outport
  wires:
  Bit Slice/1 -> Switch/2
  signof/1 -> Bit Slice/1
  base/1 -> Switch/1, Unary Minus/1
  Switch/1 -> out/1
  Unary Minus/1 -> Switch/3

== system all_together_simu_v2/Gradient Filter/CordicAtan2/Iteration_6/X_Logic ==
  xo : Inport
  yo : Inport  Port=2
  Add2 : Sum
  Bit Shift : hdlsllib/Logic and Bit Operations/Bit Shift  mode=Shift Right Arithmetic  N=5
  zsign : Subsystem
  x : Outport
  wires:
  yo/1 -> zsign/1(signof), Bit Shift/1
  Bit Shift/1 -> zsign/2(base)
  xo/1 -> Add2/1
  Add2/1 -> x/1
  zsign/1(out) -> Add2/2  "xo"

== system all_together_simu_v2/Gradient Filter/CordicAtan2/Iteration_6/Y_Logic ==
  xo : Inport
  yo : Inport  Port=2
  Add1 : Sum  OutDataTypeStr=fixdt(1,16,18)
  Bit Shift : hdlsllib/Logic and Bit Operations/Bit Shift  mode=Shift Right Arithmetic  N=5
  n_zsign : Subsystem
  y : Outport
  wires:
  Bit Shift/1 -> n_zsign/2(base)
  n_zsign/1(out) -> Add1/2
  Add1/1 -> y/1
  xo/1 -> Bit Shift/1
  yo/1 -> n_zsign/1(signof), Add1/1

== system all_together_simu_v2/Gradient Filter/CordicAtan2/Iteration_6/n_zsign ==
  signof : Inport
  base : Inport  Port=2
  Bit Slice : hdlsllib/Logic and Bit Operations/Bit Slice  lidx=15  ridx=15
      settings: SourceProductBaseCode=SL
  Switch : Switch  Criteria=u2 > Threshold
  Unary Minus : UnaryMinus
  out : Outport
  wires:
  Bit Slice/1 -> Switch/2
  signof/1 -> Bit Slice/1
  base/1 -> Switch/1, Unary Minus/1
  Switch/1 -> out/1
  Unary Minus/1 -> Switch/3

== system all_together_simu_v2/Gradient Filter/CordicAtan2/Iteration_7/X_Logic ==
  xo : Inport
  yo : Inport  Port=2
  Add2 : Sum
  Bit Shift : hdlsllib/Logic and Bit Operations/Bit Shift  mode=Shift Right Arithmetic  N=6
  zsign : Subsystem
  x : Outport
  wires:
  yo/1 -> zsign/1(signof), Bit Shift/1
  Bit Shift/1 -> zsign/2(base)
  xo/1 -> Add2/1
  Add2/1 -> x/1
  zsign/1(out) -> Add2/2  "xo"

== system all_together_simu_v2/Gradient Filter/CordicAtan2/Iteration_7/Y_Logic ==
  xo : Inport
  yo : Inport  Port=2
  Add1 : Sum  OutDataTypeStr=fixdt(1,16,19)
  Bit Shift : hdlsllib/Logic and Bit Operations/Bit Shift  mode=Shift Right Arithmetic  N=6
  n_zsign : Subsystem
  y : Outport
  wires:
  Bit Shift/1 -> n_zsign/2(base)
  n_zsign/1(out) -> Add1/2
  Add1/1 -> y/1
  xo/1 -> Bit Shift/1
  yo/1 -> n_zsign/1(signof), Add1/1

== system all_together_simu_v2/Gradient Filter/CordicAtan2/Iteration_7/n_zsign ==
  signof : Inport
  base : Inport  Port=2
  Bit Slice : hdlsllib/Logic and Bit Operations/Bit Slice  lidx=15  ridx=15
      settings: SourceProductBaseCode=SL
  Switch : Switch  Criteria=u2 > Threshold
  Unary Minus : UnaryMinus
  out : Outport
  wires:
  Bit Slice/1 -> Switch/2
  signof/1 -> Bit Slice/1
  base/1 -> Switch/1, Unary Minus/1
  Switch/1 -> out/1
  Unary Minus/1 -> Switch/3

== system all_together_simu_v2/Gradient Filter/CordicAtan2/Iteration_8/X_Logic ==
  xo : Inport
  yo : Inport  Port=2
  Add2 : Sum
  Bit Shift : hdlsllib/Logic and Bit Operations/Bit Shift  mode=Shift Right Arithmetic  N=7
  zsign : Subsystem
  x : Outport
  wires:
  yo/1 -> zsign/1(signof), Bit Shift/1
  Bit Shift/1 -> zsign/2(base)
  xo/1 -> Add2/1
  Add2/1 -> x/1
  zsign/1(out) -> Add2/2  "xo"

== system all_together_simu_v2/Gradient Filter/CordicAtan2/Iteration_8/Y_Logic ==
  xo : Inport
  yo : Inport  Port=2
  Add1 : Sum  OutDataTypeStr=fixdt(1,16,20)
  Bit Shift : hdlsllib/Logic and Bit Operations/Bit Shift  mode=Shift Right Arithmetic  N=7
  n_zsign : Subsystem
  y : Outport
  wires:
  Bit Shift/1 -> n_zsign/2(base)
  n_zsign/1(out) -> Add1/2
  Add1/1 -> y/1
  xo/1 -> Bit Shift/1
  yo/1 -> n_zsign/1(signof), Add1/1

== system all_together_simu_v2/Gradient Filter/CordicAtan2/Iteration_8/n_zsign ==
  signof : Inport
  base : Inport  Port=2
  Bit Slice : hdlsllib/Logic and Bit Operations/Bit Slice  lidx=15  ridx=15
      settings: SourceProductBaseCode=SL
  Switch : Switch  Criteria=u2 > Threshold
  Unary Minus : UnaryMinus
  out : Outport
  wires:
  Bit Slice/1 -> Switch/2
  signof/1 -> Bit Slice/1
  base/1 -> Switch/1, Unary Minus/1
  Switch/1 -> out/1
  Unary Minus/1 -> Switch/3

== system all_together_simu_v2/Gradient Filter/CordicAtan2/Iteration_9/X_Logic ==
  xo : Inport
  yo : Inport  Port=2
  Add2 : Sum
  Bit Shift : hdlsllib/Logic and Bit Operations/Bit Shift  mode=Shift Right Arithmetic  N=8
  zsign : Subsystem
  x : Outport
  wires:
  yo/1 -> zsign/1(signof), Bit Shift/1
  Bit Shift/1 -> zsign/2(base)
  xo/1 -> Add2/1
  Add2/1 -> x/1
  zsign/1(out) -> Add2/2  "xo"

== system all_together_simu_v2/Gradient Filter/CordicAtan2/Iteration_9/Y_Logic ==
  xo : Inport
  yo : Inport  Port=2
  Add1 : Sum  OutDataTypeStr=fixdt(1,16,21)
  Bit Shift : hdlsllib/Logic and Bit Operations/Bit Shift  mode=Shift Right Arithmetic  N=8
  n_zsign : Subsystem
  y : Outport
  wires:
  Bit Shift/1 -> n_zsign/2(base)
  n_zsign/1(out) -> Add1/2
  Add1/1 -> y/1
  xo/1 -> Bit Shift/1
  yo/1 -> n_zsign/1(signof), Add1/1

== system all_together_simu_v2/Gradient Filter/CordicAtan2/Iteration_9/n_zsign ==
  signof : Inport
  base : Inport  Port=2
  Bit Slice : hdlsllib/Logic and Bit Operations/Bit Slice  lidx=15  ridx=15
      settings: SourceProductBaseCode=SL
  Switch : Switch  Criteria=u2 > Threshold
  Unary Minus : UnaryMinus
  out : Outport
  wires:
  Bit Slice/1 -> Switch/2
  signof/1 -> Bit Slice/1
  base/1 -> Switch/1, Unary Minus/1
  Switch/1 -> out/1
  Unary Minus/1 -> Switch/3

== system all_together_simu_v2/Gradient Filter/CordicAtan2/Setup_Stage/n_zsign ==
  signof : Inport
  base : Inport  Port=2
  Bit Slice : hdlsllib/Logic and Bit Operations/Bit Slice  lidx=15  ridx=15
      settings: SourceProductBaseCode=SL
  Switch : Switch  Criteria=u2 > Threshold
  Unary Minus : UnaryMinus
  out : Outport
  wires:
  Bit Slice/1 -> Switch/2
  signof/1 -> Bit Slice/1
  base/1 -> Switch/1, Unary Minus/1
  Switch/1 -> out/1
  Unary Minus/1 -> Switch/3

== system all_together_simu_v2/Gradient Filter/CordicAtan2/Setup_Stage/n_zsign1 ==
  signof : Inport
  base : Inport  Port=2
  Bit Slice : hdlsllib/Logic and Bit Operations/Bit Slice  lidx=15  ridx=15
      settings: SourceProductBaseCode=SL
  Switch : Switch  Criteria=u2 > Threshold
  Unary Minus : UnaryMinus
  out : Outport
  wires:
  Bit Slice/1 -> Switch/2
  signof/1 -> Bit Slice/1
  base/1 -> Switch/1, Unary Minus/1
  Switch/1 -> out/1
  Unary Minus/1 -> Switch/3

== system all_together_simu_v2/Gradient Filter/CordicAtan2/Setup_Stage/n_zsign2 ==
  signof : Inport
  base : Inport  Port=2
  Bit Slice : hdlsllib/Logic and Bit Operations/Bit Slice  lidx=15  ridx=15
      settings: SourceProductBaseCode=SL
  Switch : Switch  Criteria=u2 > Threshold
  Unary Minus : UnaryMinus
  out : Outport
  wires:
  Bit Slice/1 -> Switch/2
  signof/1 -> Bit Slice/1
  base/1 -> Switch/1, Unary Minus/1
  Switch/1 -> out/1
  Unary Minus/1 -> Switch/3

== system all_together_simu_v2/Gradient Filter/CordicAtan2/Setup_Stage/zsign ==
  signof : Inport
  base : Inport  Port=2
  Bit Slice : hdlsllib/Logic and Bit Operations/Bit Slice  lidx=15  ridx=15
      settings: SourceProductBaseCode=SL
  Switch : Switch  Criteria=u2 > Threshold
  Unary Minus : UnaryMinus
  out : Outport
  wires:
  signof/1 -> Bit Slice/1
  Bit Slice/1 -> Switch/2
  base/1 -> Switch/3, Unary Minus/1
  Switch/1 -> out/1
  Unary Minus/1 -> Switch/1

== system all_together_simu_v2/Gradient Filter/Ix//Iy Filters/Ix Filter/Filter ==
  data_in : Inport
  Enable : EnablePort
  Row Filter2 : Subsystem
  Terminator : Terminator
  Terminator1 : Terminator
  slicer : Subsystem
  data_out : Outport
  wires:
  data_in/1 -> slicer/1(data_in)
  slicer/2(Row2) -> Row Filter2/1(data_in)
  Row Filter2/1(data_out) -> data_out/1
  slicer/1(Row1) -> Terminator/1
  slicer/3(Row3) -> Terminator1/1

== system all_together_simu_v2/Gradient Filter/Ix//Iy Filters/Iy Filter/Filter ==
  data_in : Inport
  Enable : EnablePort
  Constant : Constant  Value=0  OutDataTypeStr=Inherit: Inherit via back propagation  SampleTime=-1
  Mux : Mux  Inputs=3
  Row Filter1 : Subsystem
  Row Filter3 : Subsystem
  Terminator : Terminator
  Verticle Filter : Subsystem
  slicer : Subsystem
  data_out : Outport
  wires:
  Row Filter1/1(data_out) -> Mux/1
  slicer/1(Row1) -> Row Filter1/1(data_in)
  data_in/1 -> slicer/1(data_in)
  slicer/2(Row2) -> Terminator/1
  slicer/3(Row3) -> Row Filter3/1(data_in)
  Mux/1 -> Verticle Filter/1(data_in)
  Verticle Filter/1(data_out) -> data_out/1
  Row Filter3/1(data_out) -> Mux/3
  Constant/1 -> Mux/2

== system all_together_simu_v2/Gradient Filter/CordicAtan2/Iteration_10/X_Logic/zsign ==
  signof : Inport
  base : Inport  Port=2
  Bit Slice : hdlsllib/Logic and Bit Operations/Bit Slice  lidx=15  ridx=15
      settings: SourceProductBaseCode=SL
  Switch : Switch  Criteria=u2 > Threshold
  Unary Minus : UnaryMinus
  out : Outport
  wires:
  signof/1 -> Bit Slice/1
  Bit Slice/1 -> Switch/2
  base/1 -> Switch/3, Unary Minus/1
  Switch/1 -> out/1
  Unary Minus/1 -> Switch/1

== system all_together_simu_v2/Gradient Filter/CordicAtan2/Iteration_10/Y_Logic/n_zsign ==
  signof : Inport
  base : Inport  Port=2
  Bit Slice : hdlsllib/Logic and Bit Operations/Bit Slice  lidx=15  ridx=15
      settings: SourceProductBaseCode=SL
  Switch : Switch  Criteria=u2 > Threshold
  Unary Minus : UnaryMinus
  out : Outport
  wires:
  Bit Slice/1 -> Switch/2
  signof/1 -> Bit Slice/1
  base/1 -> Switch/1, Unary Minus/1
  Switch/1 -> out/1
  Unary Minus/1 -> Switch/3

== system all_together_simu_v2/Gradient Filter/CordicAtan2/Iteration_2/X_Logic/zsign1 ==
  signof : Inport
  base : Inport  Port=2
  Bit Slice : hdlsllib/Logic and Bit Operations/Bit Slice  lidx=15  ridx=15
      settings: SourceProductBaseCode=SL
  Switch : Switch  Criteria=u2 > Threshold
  Unary Minus : UnaryMinus
  out : Outport
  wires:
  signof/1 -> Bit Slice/1
  Bit Slice/1 -> Switch/2
  base/1 -> Switch/3, Unary Minus/1
  Switch/1 -> out/1
  Unary Minus/1 -> Switch/1

== system all_together_simu_v2/Gradient Filter/CordicAtan2/Iteration_2/Y_Logic/n_zsign ==
  signof : Inport
  base : Inport  Port=2
  Bit Slice : hdlsllib/Logic and Bit Operations/Bit Slice  lidx=15  ridx=15
      settings: SourceProductBaseCode=SL
  Switch : Switch  Criteria=u2 > Threshold
  Unary Minus : UnaryMinus
  out : Outport
  wires:
  Bit Slice/1 -> Switch/2
  signof/1 -> Bit Slice/1
  base/1 -> Switch/1, Unary Minus/1
  Switch/1 -> out/1
  Unary Minus/1 -> Switch/3

== system all_together_simu_v2/Gradient Filter/CordicAtan2/Iteration_3/X_Logic/zsign ==
  signof : Inport
  base : Inport  Port=2
  Bit Slice : hdlsllib/Logic and Bit Operations/Bit Slice  lidx=15  ridx=15
      settings: SourceProductBaseCode=SL
  Switch : Switch  Criteria=u2 > Threshold
  Unary Minus : UnaryMinus
  out : Outport
  wires:
  signof/1 -> Bit Slice/1
  Bit Slice/1 -> Switch/2
  base/1 -> Switch/3, Unary Minus/1
  Switch/1 -> out/1
  Unary Minus/1 -> Switch/1

== system all_together_simu_v2/Gradient Filter/CordicAtan2/Iteration_3/Y_Logic/n_zsign ==
  signof : Inport
  base : Inport  Port=2
  Bit Slice : hdlsllib/Logic and Bit Operations/Bit Slice  lidx=15  ridx=15
      settings: SourceProductBaseCode=SL
  Switch : Switch  Criteria=u2 > Threshold
  Unary Minus : UnaryMinus
  out : Outport
  wires:
  Bit Slice/1 -> Switch/2
  signof/1 -> Bit Slice/1
  base/1 -> Switch/1, Unary Minus/1
  Switch/1 -> out/1
  Unary Minus/1 -> Switch/3

== system all_together_simu_v2/Gradient Filter/CordicAtan2/Iteration_4/X_Logic/zsign ==
  signof : Inport
  base : Inport  Port=2
  Bit Slice : hdlsllib/Logic and Bit Operations/Bit Slice  lidx=15  ridx=15
      settings: SourceProductBaseCode=SL
  Switch : Switch  Criteria=u2 > Threshold
  Unary Minus : UnaryMinus
  out : Outport
  wires:
  signof/1 -> Bit Slice/1
  Bit Slice/1 -> Switch/2
  base/1 -> Switch/3, Unary Minus/1
  Switch/1 -> out/1
  Unary Minus/1 -> Switch/1

== system all_together_simu_v2/Gradient Filter/CordicAtan2/Iteration_4/Y_Logic/n_zsign ==
  signof : Inport
  base : Inport  Port=2
  Bit Slice : hdlsllib/Logic and Bit Operations/Bit Slice  lidx=15  ridx=15
      settings: SourceProductBaseCode=SL
  Switch : Switch  Criteria=u2 > Threshold
  Unary Minus : UnaryMinus
  out : Outport
  wires:
  Bit Slice/1 -> Switch/2
  signof/1 -> Bit Slice/1
  base/1 -> Switch/1, Unary Minus/1
  Switch/1 -> out/1
  Unary Minus/1 -> Switch/3

== system all_together_simu_v2/Gradient Filter/CordicAtan2/Iteration_5/X_Logic/zsign ==
  signof : Inport
  base : Inport  Port=2
  Bit Slice : hdlsllib/Logic and Bit Operations/Bit Slice  lidx=15  ridx=15
      settings: SourceProductBaseCode=SL
  Switch : Switch  Criteria=u2 > Threshold
  Unary Minus : UnaryMinus
  out : Outport
  wires:
  signof/1 -> Bit Slice/1
  Bit Slice/1 -> Switch/2
  base/1 -> Switch/3, Unary Minus/1
  Switch/1 -> out/1
  Unary Minus/1 -> Switch/1

== system all_together_simu_v2/Gradient Filter/CordicAtan2/Iteration_5/Y_Logic/n_zsign ==
  signof : Inport
  base : Inport  Port=2
  Bit Slice : hdlsllib/Logic and Bit Operations/Bit Slice  lidx=15  ridx=15
      settings: SourceProductBaseCode=SL
  Switch : Switch  Criteria=u2 > Threshold
  Unary Minus : UnaryMinus
  out : Outport
  wires:
  Bit Slice/1 -> Switch/2
  signof/1 -> Bit Slice/1
  base/1 -> Switch/1, Unary Minus/1
  Switch/1 -> out/1
  Unary Minus/1 -> Switch/3

== system all_together_simu_v2/Gradient Filter/CordicAtan2/Iteration_6/X_Logic/zsign ==
  signof : Inport
  base : Inport  Port=2
  Bit Slice : hdlsllib/Logic and Bit Operations/Bit Slice  lidx=15  ridx=15
      settings: SourceProductBaseCode=SL
  Switch : Switch  Criteria=u2 > Threshold
  Unary Minus : UnaryMinus
  out : Outport
  wires:
  signof/1 -> Bit Slice/1
  Bit Slice/1 -> Switch/2
  base/1 -> Switch/3, Unary Minus/1
  Switch/1 -> out/1
  Unary Minus/1 -> Switch/1
